simulink model "teleoperation"  (R2018a)
settings: Solver=ode45  StartTime=0.0  StopTime=10  RelTol=1e-3
values from neighbouring files (symbols this model uses):
  B_e = 0.01    [simulinkTeleop.m]
  B_h = humanDamp*armL    (= 0.4)    [simulinkTeleop.m]
  B_v = 0.15    [simulinkTeleop.m]
  J_m = 0.0005    [simulinkTeleop.m]
  J_s = 0.0005    [simulinkTeleop.m]
  J_v = 0.0    (= 0)    [simulinkTeleop.m]
  K_e = 1000    [simulinkTeleop.m]
  K_h = humanStiff*armL    (= 20)    [simulinkTeleop.m]
  K_v = 100.0    (= 100)    [simulinkTeleop.m]
  theta_s_contact = -0.0    (= 0)    [simulinkTeleop.m]
libraries: cstblocks x5, simulink x1
settings Model: Creator=dinies33  LastModifiedBy=giuseppe

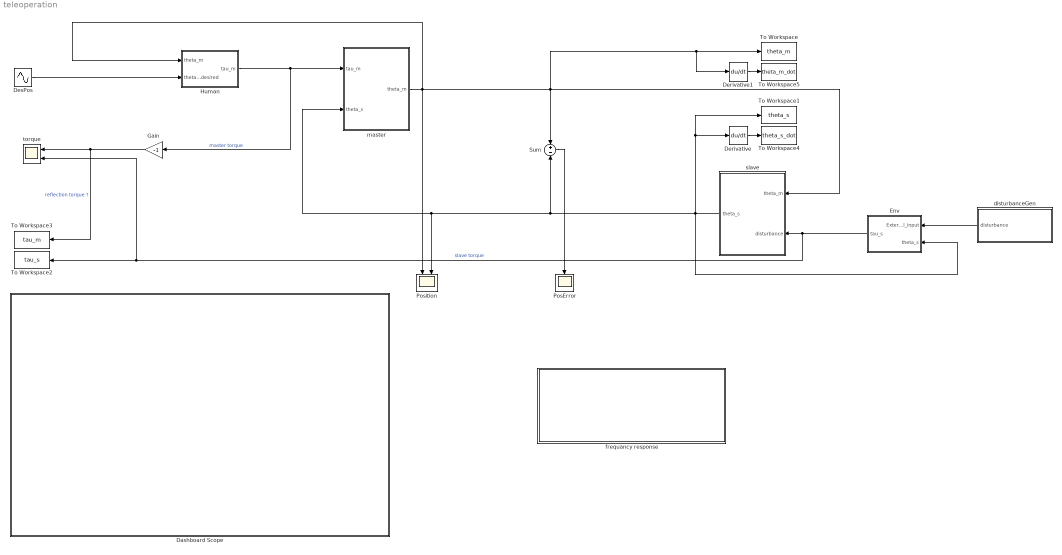
== system teleoperation ==
  Dashboard Scope : Subsystem  DialogController=hmiCreateDDGDialog  IsWebBlock=on  mask(MWDashboardBlock){webBlockId=d953983e-eab8-4310-ba24-9145e9f5b59c, webBlockType=sdiscope, ShowInitialText=on, HMISrcModelName=teleoperation}
      mask prompts: webBlockId "WebBlock Id"; webBlockType "WebBlock Type"; HMISrcModelName "Source Model"
      mask help: SimulinkHMI:dialogs:HMIScopeDialogDesc
      mask Help: helpview([docroot '/mapfiles/simulink.map'], 'hmi_scope')
      mask Display:
      | if strcmp(get_param(bdroot(gcb),'BlockDiagramType'), 'library')
      |     image([(matlabroot) '/toolbox/simulink/hmi/icons/DashboardScope.png']);
      | end
  Derivative : Derivative  CoefficientInTFapproximation=0
  Derivative1 : Derivative  CoefficientInTFapproximation=0
  DesPos : Sin  Amplitude=0.18  Frequency=0.11*(6.28)  SampleTime=0
  Env : Subsystem
  Gain : Gain  Gain=-1
  Human : Subsystem
  PosError : Scope
  Position : Scope  NumInputPorts=2
  Sum : Sum  Inputs=+-
  To Workspace : ToWorkspace  VariableName=theta_m  SampleTime=-1
  To Workspace1 : ToWorkspace  VariableName=theta_s  SampleTime=-1
  To Workspace2 : ToWorkspace  VariableName=tau_s  SampleTime=-1
  To Workspace3 : ToWorkspace  VariableName=tau_m  SampleTime=-1
  To Workspace4 : ToWorkspace  VariableName=theta_s_dot  SampleTime=-1
  To Workspace5 : ToWorkspace  VariableName=theta_m_dot  SampleTime=-1
  disturbanceGen : Subsystem
  frequancy response : Subsystem
  master : Subsystem
  "slave " : Subsystem
  torque : Scope  NumInputPorts=2
  wires:
  Env/1("tau_s ") -> torque/2, To Workspace2/1, "slave "/2(disturbance)  "slave torque"
  DesPos/1 -> Human/2(theta_desired)
  master/1(theta_m) -> Derivative1/1, To Workspace/1, "slave "/1("theta_m "), Sum/1, Human/1(theta_m), Position/1
  Human/1(tau_m) -> Gain/1, master/1(tau_m)  "master torque"
  "slave "/1(theta_s) -> Derivative/1, To Workspace1/1, Sum/2, master/2(theta_s), Position/2, Env/2(theta_s)
  Gain/1 -> To Workspace3/1, torque/1  "reflection torque ?"
  Sum/1 -> PosError/1
  Derivative1/1 -> To Workspace5/1
  Derivative/1 -> To Workspace4/1
  disturbanceGen/1(disturbance) -> Env/1(External_input)

== system teleoperation/Dashboard Scope ==

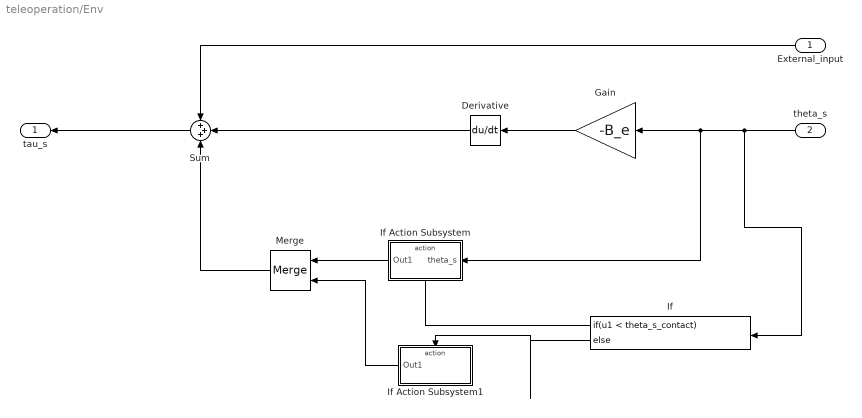
== system teleoperation/Env ==
  External_input : Inport
  theta_s : Inport  Port=2
  Derivative : Derivative  CoefficientInTFapproximation=0
  Gain : Gain  Gain=-B_e
  If : If  IfExpression=u1 < theta_s_contact
  If Action Subsystem : Subsystem  TreatAsAtomicUnit=on
  If Action Subsystem1 : Subsystem  TreatAsAtomicUnit=on
  Merge : Merge
  Sum : Sum  Inputs=+++
  "tau_s " : Outport
  wires:
  External_input/1 -> Sum/1
  theta_s/1 -> If/1, If Action Subsystem/1(theta_s), Gain/1
  Gain/1 -> Derivative/1
  Derivative/1 -> Sum/2
  Sum/1 -> "tau_s "/1
  If/2 -> If Action Subsystem1/Action
  If/1 -> If Action Subsystem/Action
  If Action Subsystem1/1(Out1) -> Merge/2
  If Action Subsystem/1(Out1) -> Merge/1
  Merge/1 -> Sum/3

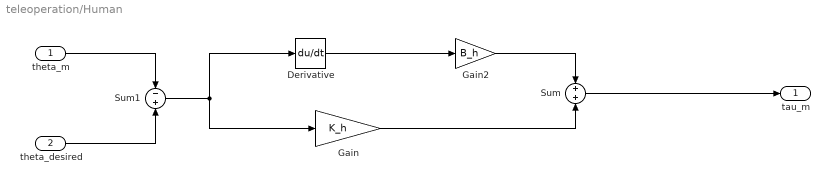
== system teleoperation/Human ==
  theta_m : Inport
  theta_desired : Inport  Port=2
  Derivative : Derivative  CoefficientInTFapproximation=0
  Gain : Gain  Gain=K_h
  Gain2 : Gain  Gain=B_h
  Sum : Sum  Inputs=+|+
  Sum1 : Sum  Inputs=-|+
  tau_m : Outport
  wires:
  Derivative/1 -> Gain2/1
  theta_m/1 -> Sum1/1
  theta_desired/1 -> Sum1/2
  Sum1/1 -> Derivative/1, Gain/1
  Gain2/1 -> Sum/1
  Gain/1 -> Sum/2
  Sum/1 -> tau_m/1

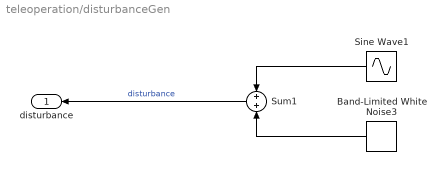
== system teleoperation/disturbanceGen ==
  Band-Limited White Noise3 : simulink/Sources/Band-Limited White Noise  Cov=0.001  Ts=1/20  seed=[12345]
  Sine Wave1 : Sin  Amplitude=0.015  Frequency=20*(6.28)  SampleTime=0
  Sum1 : Sum
  disturbance : Outport
  wires:
  Band-Limited White Noise3/1 -> Sum1/2
  Sine Wave1/1 -> Sum1/1
  Sum1/1 -> disturbance/1  "disturbance"

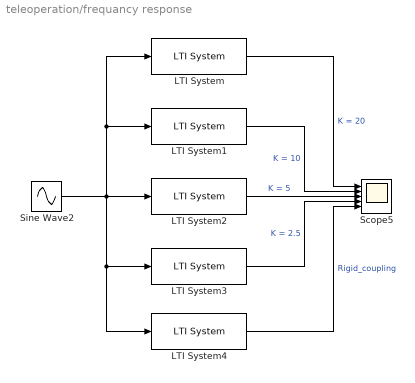
== system teleoperation/frequancy response ==
  LTI System : cstblocks/LTI System  sys=set_1  IC=[]
  LTI System1 : cstblocks/LTI System  sys=set_2  IC=[]
  LTI System2 : cstblocks/LTI System  sys=set_3  IC=[]
  LTI System3 : cstblocks/LTI System  sys=set_4  IC=[]
  LTI System4 : cstblocks/LTI System  sys=rigid  IC=[]
  Scope5 : Scope  NumInputPorts=5
  Sine Wave2 : Sin  Amplitude=0.1  Frequency=10*(6.28)  SampleTime=0
  wires:
  LTI System4/1 -> Scope5/5  "Rigid_coupling"
  LTI System3/1 -> Scope5/4  "K = 2.5"
  LTI System/1 -> Scope5/1  "K = 20"
  LTI System1/1 -> Scope5/2  "K = 10"
  Sine Wave2/1 -> LTI System4/1, LTI System3/1, LTI System2/1, LTI System1/1, LTI System/1
  LTI System2/1 -> Scope5/3  "K = 5"

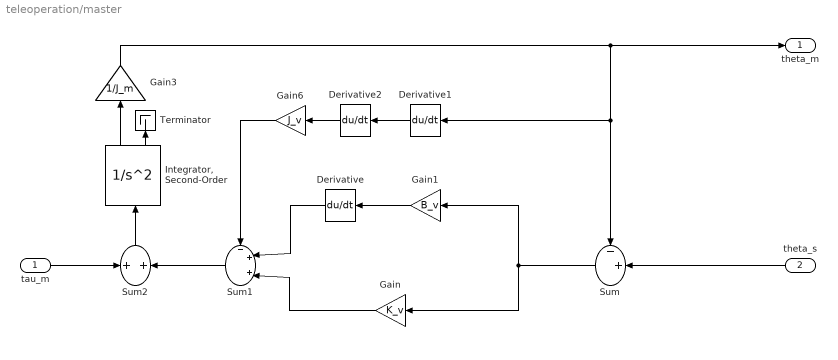
== system teleoperation/master ==
  tau_m : Inport
  theta_s : Inport  Port=2
  Derivative : Derivative  CoefficientInTFapproximation=0
  Derivative1 : Derivative  CoefficientInTFapproximation=0
  Derivative2 : Derivative  CoefficientInTFapproximation=0
  Gain : Gain  Gain=K_v
  Gain1 : Gain  Gain=B_v
  Gain3 : Gain  Gain=1/J_m
  Gain6 : Gain  Gain=J_v
  "Integrator, Second-Order" : SecondOrderIntegrator  ICX=0
  Sum : Sum  Inputs=-+|
  Sum1 : Sum  Inputs=-++|
  Sum2 : Sum  Inputs=+|+
  Terminator : Terminator
  theta_m : Outport
  wires:
  Derivative1/1 -> Derivative2/1
  "Integrator, Second-Order"/1 -> Gain3/1
  theta_s/1 -> Sum/2
  Gain/1 -> Sum1/3
  Sum/1 -> Gain/1, Gain1/1
  Sum1/1 -> Sum2/2
  Derivative2/1 -> Gain6/1
  Derivative/1 -> Sum1/2
  Gain6/1 -> Sum1/1
  Gain1/1 -> Derivative/1
  Sum2/1 -> "Integrator, Second-Order"/1
  tau_m/1 -> Sum2/1
  Gain3/1 -> theta_m/1, Derivative1/1, Sum/1
  "Integrator, Second-Order"/2 -> Terminator/1

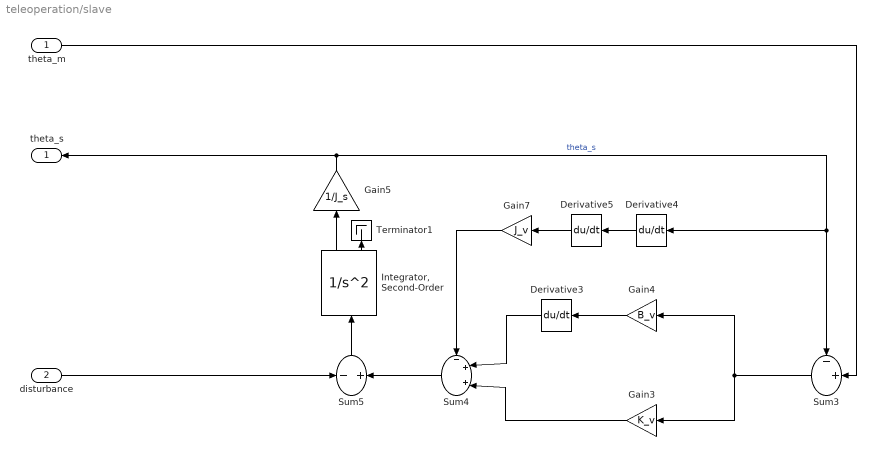
== system teleoperation/slave  ==
  "theta_m " : Inport
  disturbance : Inport  Port=2
  Derivative3 : Derivative  CoefficientInTFapproximation=0
  Derivative4 : Derivative  CoefficientInTFapproximation=0
  Derivative5 : Derivative  CoefficientInTFapproximation=0
  Gain3 : Gain  Gain=K_v
  Gain4 : Gain  Gain=B_v
  Gain5 : Gain  Gain=1/J_s
  Gain7 : Gain  Gain=J_v
  "Integrator, Second-Order" : SecondOrderIntegrator  ICX=0
  Sum3 : Sum  Inputs=-+|
  Sum4 : Sum  Inputs=-++|
  Sum5 : Sum  Inputs=-|+
  Terminator1 : Terminator
  theta_s : Outport
  wires:
  Sum5/1 -> "Integrator, Second-Order"/1
  Gain7/1 -> Sum4/1
  "Integrator, Second-Order"/1 -> Gain5/1
  Derivative5/1 -> Gain7/1
  Sum4/1 -> Sum5/2
  Derivative3/1 -> Sum4/2
  Gain4/1 -> Derivative3/1
  Gain5/1 -> Derivative4/1, Sum3/1, theta_s/1  "theta_s"
  Gain3/1 -> Sum4/3
  "theta_m "/1 -> Sum3/2
  Sum3/1 -> Gain3/1, Gain4/1
  Derivative4/1 -> Derivative5/1
  disturbance/1 -> Sum5/1
  "Integrator, Second-Order"/2 -> Terminator1/1

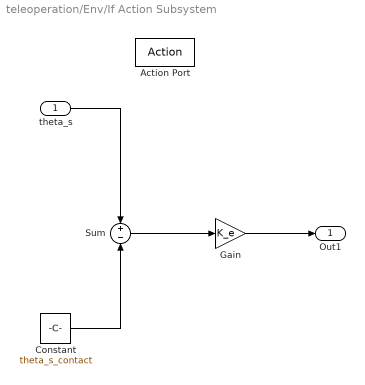
== system teleoperation/Env/If Action Subsystem ==
  theta_s : Inport
  Action Port : ActionPort  ActionType=then
  Constant : Constant  Value=theta_s_contact
  Gain : Gain  Gain=K_e
  Sum : Sum  Inputs=+-
  Out1 : Outport
  wires:
  theta_s/1 -> Sum/1
  Constant/1 -> Sum/2
  Sum/1 -> Gain/1
  Gain/1 -> Out1/1

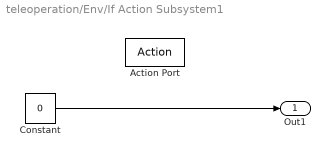
== system teleoperation/Env/If Action Subsystem1 ==
  Action Port : ActionPort  ActionType=else
  Constant : Constant  Value=0
  Out1 : Outport
  wires:
  Constant/1 -> Out1/1
